simulink model "hw2c"  (R2017a)
settings: Solver=VariableStepAuto  StartTime=0.0  StopTime=10.0  RelTol=1e-3
settings Model: Creator=Soutrik  LastModifiedBy=Soutrik

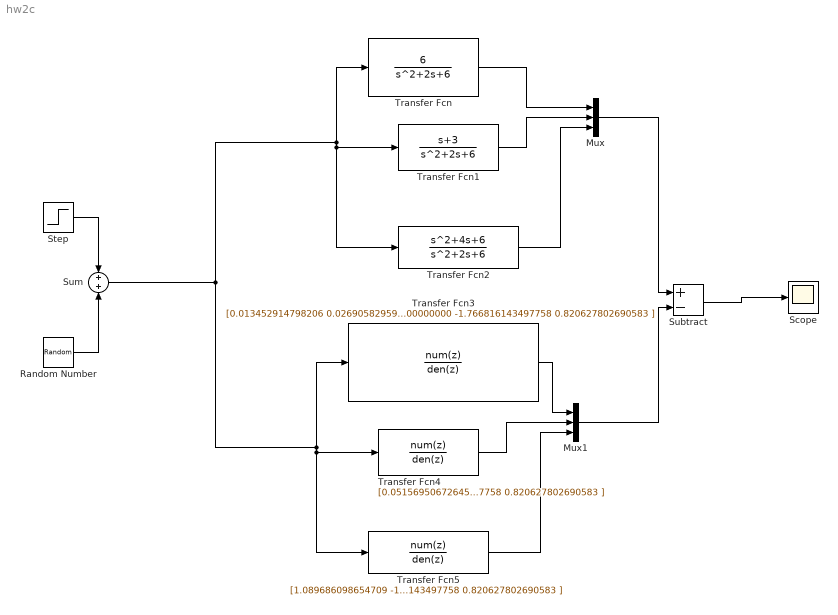
== system hw2c ==
  Mux : Mux  Inputs=3
  Mux1 : Mux  Inputs=3
  Random Number : RandomNumber  Variance=0.01  SampleTime=0.1
  Scope : Scope
  Step : Step  SampleTime=0.1
  Subtract : Sum  Inputs=+-
  Sum : Sum
  Transfer Fcn : TransferFcn  Numerator=[6]  Denominator=[1 2 6]
  Transfer Fcn1 : TransferFcn  Numerator=[1 3]  Denominator=[1 2 6]
  Transfer Fcn2 : TransferFcn  Numerator=[1 4 6]  Denominator=[1 2 6]
  Transfer Fcn3 : DiscreteTransferFcn  Numerator=[0.013452914798206 0.026905829596413 0.013452914798206 ]  Denominator=[1.000000000000000 -1.766816143497758 0.820627802690583 ]  SampleTime=0.10000000000000001
  Transfer Fcn4 : DiscreteTransferFcn  Numerator=[0.051569506726457 0.013452914798206 -0.038116591928251 ]  Denominator=[1.000000000000000 -1.766816143497758 0.820627802690583 ]  SampleTime=0.10000000000000001
  Transfer Fcn5 : DiscreteTransferFcn  Numerator=[1.089686098654709 -1.766816143497758 0.730941704035875 ]  Denominator=[1.000000000000000 -1.766816143497758 0.820627802690583 ]  SampleTime=0.10000000000000001
  wires:
  Mux/1 -> Subtract/1
  Mux1/1 -> Subtract/2
  Sum/1 -> Transfer Fcn3/1, Transfer Fcn4/1, Transfer Fcn5/1, Transfer Fcn2/1, Transfer Fcn1/1, Transfer Fcn/1
  Transfer Fcn3/1 -> Mux1/1
  Transfer Fcn4/1 -> Mux1/2
  Transfer Fcn1/1 -> Mux/2
  Transfer Fcn2/1 -> Mux/3
  Transfer Fcn/1 -> Mux/1
  Transfer Fcn5/1 -> Mux1/3
  Random Number/1 -> Sum/2
  Step/1 -> Sum/1
  Subtract/1 -> Scope/1
